simulink model "msl_model"  (R2015a)
settings: configuration reference "config_cosim" (kept outside this file)
model workspace (MATLAB code in the model file):
  | init_msl;
undefined symbols (not defined in the file): Cx, g, Init_beta, Init_epsi, Init_m, Init_psi, Init_R, Init_theta, Init_Vm, Init_Xm, Init_Ym, Init_Zm, Is, N, rou, S
settings Model: Creator=zhang  LastModifiedBy=ericli
settings ConfigSetRef: SourceLocation=Base Workspace

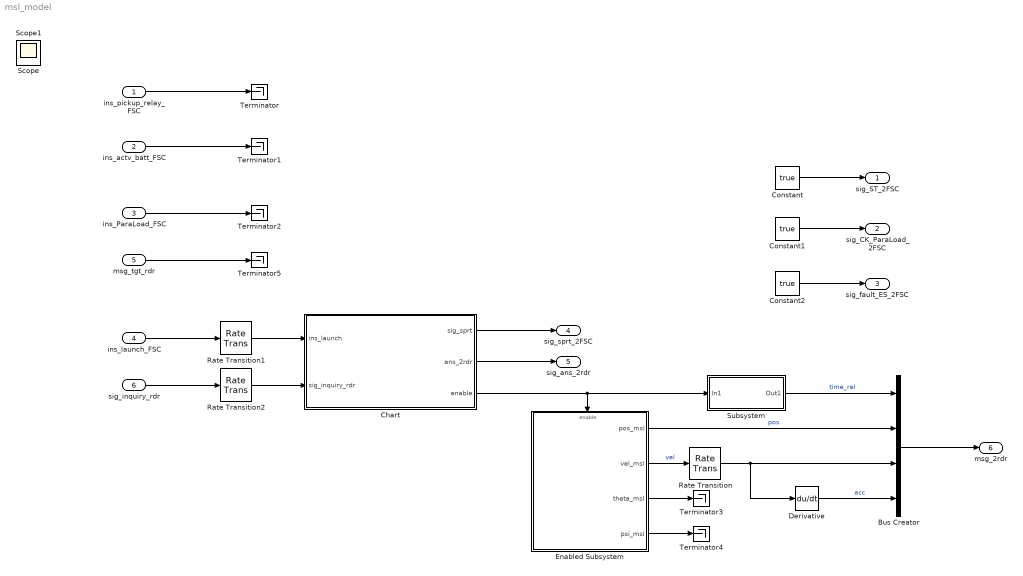
== system msl_model ==
  ins_pickup_relay_FSC : Inport  OutDataTypeStr=boolean
  ins_actv_batt_FSC : Inport  Port=2  OutDataTypeStr=boolean
  ins_ParaLoad_FSC : Inport  Port=3  OutDataTypeStr=boolean
  ins_launch_FSC : Inport  Port=4  OutDataTypeStr=boolean
  msg_tgt_rdr : Inport  Port=5  OutDataTypeStr=Bus: BusObject_msg_rdr2msl  BusOutputAsStruct=on
  sig_inquiry_rdr : Inport  Port=6  OutDataTypeStr=boolean
  Bus Creator : BusCreator  OutDataTypeStr=Bus: BusObject_msg_msl2rdr
      settings: InheritFromInputs=off
  Chart : Stateflow chart  TreatAsAtomicUnit=on
  Constant : Constant  Value=true
  Constant1 : Constant  Value=true
  Constant2 : Constant  Value=true
  Derivative : Derivative
  Enabled Subsystem : Subsystem  TreatAsAtomicUnit=on
  Rate Transition : RateTransition
  Rate Transition1 : RateTransition
  Rate Transition2 : RateTransition
  Subsystem : Subsystem
  Terminator{,1..5} (6 alike) : Terminator
  sig_ST_2FSC : Outport
  sig_CK_ParaLoad_2FSC : Outport  Port=2
  sig_fault_ES_2FSC : Outport  Port=3
  sig_sprt_2FSC : Outport  Port=4
  sig_ans_2rdr : Outport  Port=5
  msg_2rdr : Outport  Port=6  OutDataTypeStr=Bus: BusObject_msg_msl2rdr  BusOutputAsStruct=on
  Scope : Scope  NumInputPorts=3
      settings: YMin=-5~-5~-5  YMax=5~5~5
  Scope1 : Scope  NumInputPorts=3
      settings: YMin=-5~-5~-5  YMax=5~5~5
  wires:
  ins_pickup_relay_FSC/1 -> Terminator/1
  ins_actv_batt_FSC/1 -> Terminator1/1
  ins_ParaLoad_FSC/1 -> Terminator2/1
  ins_launch_FSC/1 -> Rate Transition1/1
  Chart/1(sig_sprt) -> sig_sprt_2FSC/1
  Chart/3(enable) -> Subsystem/1(In1), Enabled Subsystem/Enable
  Enabled Subsystem/4(psi_msl) -> Terminator4/1
  Enabled Subsystem/3(theta_msl) -> Terminator3/1
  Enabled Subsystem/2(vel_msl) -> Rate Transition/1  "vel"
  Constant/1 -> sig_ST_2FSC/1
  Constant1/1 -> sig_CK_ParaLoad_2FSC/1
  Constant2/1 -> sig_fault_ES_2FSC/1
  Chart/2(ans_2rdr) -> sig_ans_2rdr/1
  Enabled Subsystem/1(pos_msl) -> Bus Creator/2  "pos"
  Derivative/1 -> Bus Creator/4  "acc"
  Subsystem/1(Out1) -> Bus Creator/1  "time_rel"
  Bus Creator/1 -> msg_2rdr/1
  msg_tgt_rdr/1 -> Terminator5/1
  sig_inquiry_rdr/1 -> Rate Transition2/1
  Rate Transition/1 -> Derivative/1, Bus Creator/3
  Rate Transition1/1 -> Chart/1(ins_launch)
  Rate Transition2/1 -> Chart/2(sig_inquiry_rdr)

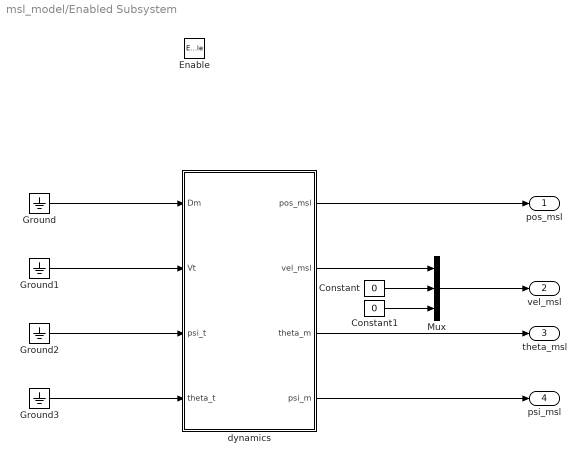
== system msl_model/Enabled Subsystem ==
  Enable : EnablePort
  Constant : Constant  Value=0
  Constant1 : Constant  Value=0
  Ground{,1..3} (4 alike) : Ground
  Mux : Mux  Inputs=3
  dynamics : Subsystem
  pos_msl : Outport
  vel_msl : Outport  Port=2
  theta_msl : Outport  Port=3
  psi_msl : Outport  Port=4
  wires:
  Ground/1 -> dynamics/1(Dm)
  Ground1/1 -> dynamics/2(Vt)
  Ground2/1 -> dynamics/3(psi_t)
  Ground3/1 -> dynamics/4(theta_t)
  dynamics/1(pos_msl) -> pos_msl/1
  dynamics/3(theta_m) -> theta_msl/1
  dynamics/4(psi_m) -> psi_msl/1
  dynamics/2(vel_msl) -> Mux/1
  Mux/1 -> vel_msl/1
  Constant/1 -> Mux/2
  Constant1/1 -> Mux/3

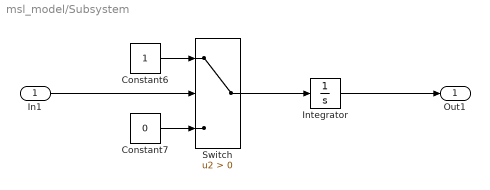
== system msl_model/Subsystem ==
  In1 : Inport
  Constant6 : Constant
  Constant7 : Constant  Value=0
  Integrator : Integrator
  Switch : Switch  Criteria=u2 > Threshold
  Out1 : Outport
  wires:
  Constant7/1 -> Switch/3
  Constant6/1 -> Switch/1
  Switch/1 -> Integrator/1
  Integrator/1 -> Out1/1
  In1/1 -> Switch/2

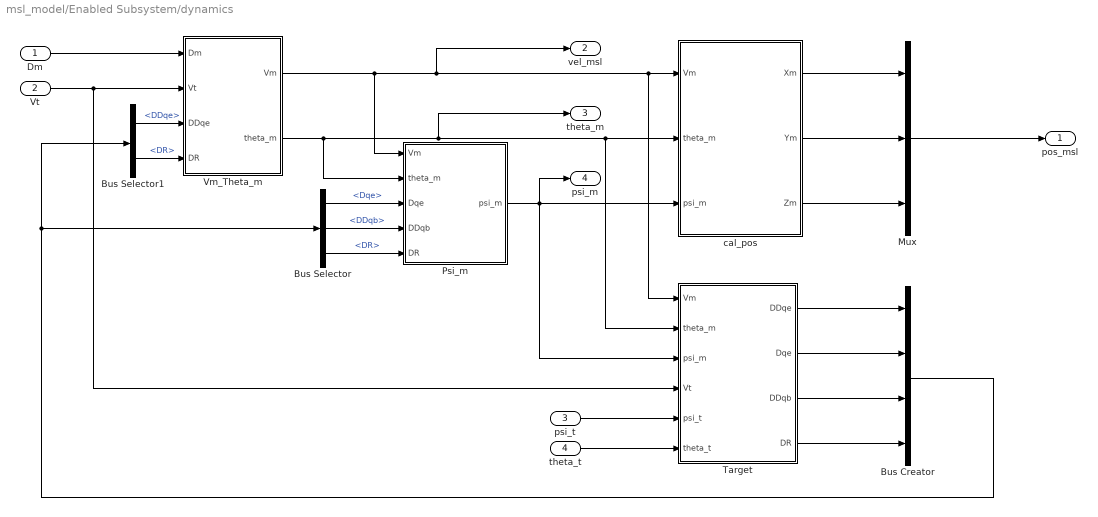
== system msl_model/Enabled Subsystem/dynamics ==
  Dm : Inport
  Vt : Inport  Port=2
  psi_t : Inport  Port=3
  theta_t : Inport  Port=4
  Bus Creator : BusCreator
  Bus Selector : BusSelector  OutputSignals=Dqe,DDqb,DR
  Bus Selector1 : BusSelector  OutputSignals=DDqe,DR
  Mux : Mux  Inputs=3
  Psi_m : Subsystem
  Target : Subsystem
  Vm_Theta_m : Subsystem
  cal_pos : Subsystem
  pos_msl : Outport
  vel_msl : Outport  Port=2
  theta_m : Outport  Port=3
  psi_m : Outport  Port=4
  wires:
  Psi_m/1(psi_m) -> psi_m/1, cal_pos/3(psi_m), Target/3(psi_m)
  Bus Selector/3 -> Psi_m/5(DR)  "<DR>"
  theta_t/1 -> Target/6(theta_t)
  Vt/1 -> Target/4(Vt), Vm_Theta_m/2(Vt)
  Target/2(Dqe) -> Bus Creator/2
  Bus Selector/1 -> Psi_m/3(Dqe)  "<Dqe>"
  Target/4(DR) -> Bus Creator/4
  cal_pos/3(Zm) -> Mux/3
  Mux/1 -> pos_msl/1
  Vm_Theta_m/1(Vm) -> Psi_m/1(Vm), vel_msl/1, cal_pos/1(Vm), Target/1(Vm)
  Bus Selector1/1 -> Vm_Theta_m/3(DDqe)  "<DDqe>"
  Bus Selector1/2 -> Vm_Theta_m/4(DR)  "<DR>"
  cal_pos/2(Ym) -> Mux/2
  Vm_Theta_m/2(theta_m) -> Psi_m/2(theta_m), theta_m/1, cal_pos/2(theta_m), Target/2(theta_m)
  Dm/1 -> Vm_Theta_m/1(Dm)
  Target/1(DDqe) -> Bus Creator/1
  psi_t/1 -> Target/5(psi_t)
  cal_pos/1(Xm) -> Mux/1
  Target/3(DDqb) -> Bus Creator/3
  Bus Selector/2 -> Psi_m/4(DDqb)  "<DDqb>"
  Bus Creator/1 -> Bus Selector/1, Bus Selector1/1

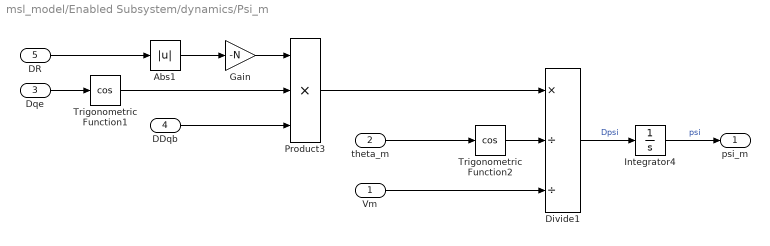
== system msl_model/Enabled Subsystem/dynamics/Psi_m ==
  Vm : Inport
  theta_m : Inport  Port=2
  Dqe : Inport  Port=3
  DDqb : Inport  Port=4
  DR : Inport  Port=5
  Abs1 : Abs
  Divide1 : Product  Inputs=*//
  Gain : Gain  Gain=-N
  Integrator4 : Integrator  InitialCondition=Init_psi
  Product3 : Product  Inputs=3
  Trigonometric Function1 : Trigonometry  Operator=cos
  Trigonometric Function2 : Trigonometry  Operator=cos
  psi_m : Outport
  wires:
  theta_m/1 -> Trigonometric Function2/1
  DR/1 -> Abs1/1
  Vm/1 -> Divide1/3
  Divide1/1 -> Integrator4/1  "Dpsi"
  Integrator4/1 -> psi_m/1  "psi"
  Trigonometric Function2/1 -> Divide1/2
  Dqe/1 -> Trigonometric Function1/1
  Product3/1 -> Divide1/1
  Abs1/1 -> Gain/1
  Gain/1 -> Product3/1
  Trigonometric Function1/1 -> Product3/2
  DDqb/1 -> Product3/3

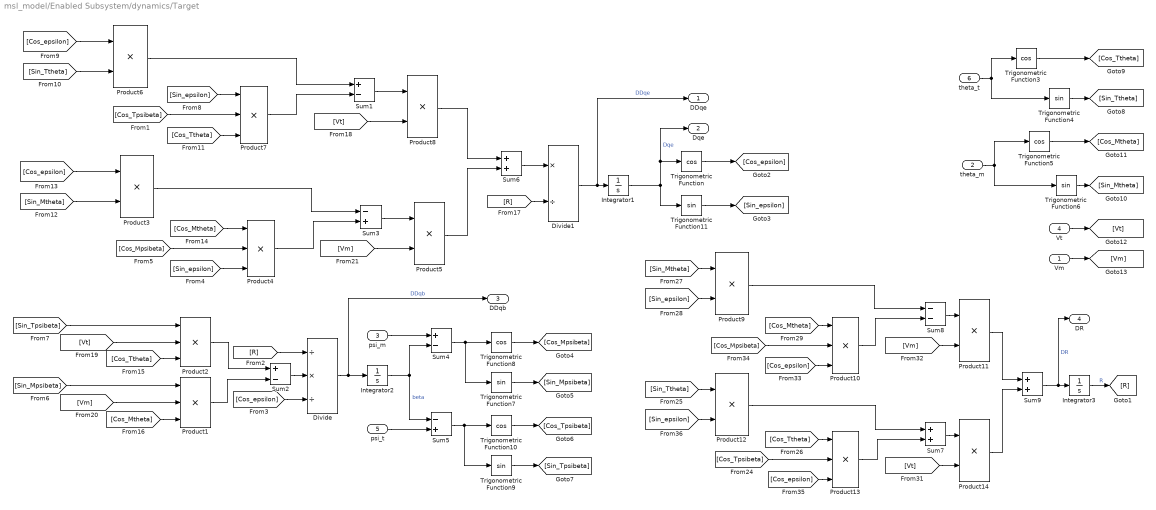
== system msl_model/Enabled Subsystem/dynamics/Target ==
  Vm : Inport
  theta_m : Inport  Port=2
  psi_m : Inport  Port=3
  Vt : Inport  Port=4
  psi_t : Inport  Port=5
  theta_t : Inport  Port=6
  Divide : Product  Inputs=/*/
  Divide1 : Product  Inputs=*/
  Integrator1 : Integrator  InitialCondition=Init_epsi
  Integrator2 : Integrator  InitialCondition=Init_beta
  Integrator3 : Integrator  InitialCondition=Init_R
  Product{1..2,4,7,10,13} (6 alike) : Product  Inputs=3
  Product{3,5..6,8..9,11..12,14} (8 alike) : Product
  Sum1 : Sum  Inputs=+-
  Sum2 : Sum  Inputs=+-
  Sum3 : Sum  Inputs=-+
  Sum4 : Sum  Inputs=+-
  Sum5 : Sum  Inputs=-+
  Sum6 : Sum
  Sum7 : Sum
  Sum8 : Sum  Inputs=--
  Sum9 : Sum
  Trigonometric Function{,3,5,8,10} (5 alike) : Trigonometry  Operator=cos
  Trigonometric Function{4,6..7,9,11} (5 alike) : Trigonometry
  DDqe : Outport
  Dqe : Outport  Port=2
  DDqb : Outport  Port=3
  DR : Outport  Port=4
  wires:
  Integrator1/1 -> Dqe/1, Trigonometric Function/1, Trigonometric Function11/1  "Dqe"
  Divide1/1 -> DDqe/1, Integrator1/1  "DDqe"
  Integrator2/1 -> Sum5/1, Sum4/2  "beta"
  Divide/1 -> DDqb/1, Integrator2/1  "DDqb"
  Integrator3/1 -> [R]  "R"
  Sum9/1 -> DR/1, Integrator3/1  "DR"
  Trigonometric Function/1 -> [Cos_epsilon]
  theta_m/1 -> Trigonometric Function5/1, Trigonometric Function6/1
  Trigonometric Function5/1 -> [Cos_Mtheta]
  Product2/1 -> Sum2/1
  Product1/1 -> Sum2/2
  [Cos_epsilon] -> Divide/3
  Product3/1 -> Sum3/1
  Product4/1 -> Sum3/2
  Sum3/1 -> Product5/1
  Trigonometric Function11/1 -> [Sin_epsilon]
  [Sin_epsilon] -> Product4/3
  psi_m/1 -> Sum4/1
  Sum4/1 -> Trigonometric Function8/1, Trigonometric Function7/1
  Trigonometric Function8/1 -> [Cos_Mpsibeta]
  Trigonometric Function7/1 -> [Sin_Mpsibeta]
  [Cos_Mpsibeta] -> Product4/2
  [Sin_Mpsibeta] -> Product1/1
  Sum5/1 -> Trigonometric Function10/1, Trigonometric Function9/1
  Trigonometric Function10/1 -> [Cos_Tpsibeta]
  Trigonometric Function9/1 -> [Sin_Tpsibeta]
  psi_t/1 -> Sum5/2
  [Sin_Tpsibeta] -> Product2/1
  Trigonometric Function6/1 -> [Sin_Mtheta]
  [Cos_Tpsibeta] -> Product7/2
  [Sin_epsilon] -> Product7/1
  [Cos_epsilon] -> Product6/1
  Product7/1 -> Sum1/2
  Product6/1 -> Sum1/1
  Sum1/1 -> Product8/1
  [Sin_Ttheta] -> Product6/2
  [Cos_Ttheta] -> Product7/3
  [Sin_Mtheta] -> Product3/2
  [Cos_Mtheta] -> Product4/1
  [Cos_Ttheta] -> Product2/3
  [Cos_Mtheta] -> Product1/3
  theta_t/1 -> Trigonometric Function4/1, Trigonometric Function3/1
  Trigonometric Function3/1 -> [Cos_Ttheta]
  Trigonometric Function4/1 -> [Sin_Ttheta]
  [Cos_epsilon] -> Product3/1
  Product5/1 -> Sum6/2
  Product8/1 -> Sum6/1
  Sum6/1 -> Divide1/1
  [R] -> Divide1/2
  Sum2/1 -> Divide/2
  [R] -> Divide/1
  [Vt] -> Product8/2
  [Vt] -> Product2/2
  [Vm] -> Product1/2
  [Vm] -> Product5/2
  Vt/1 -> [Vt]
  Vm/1 -> [Vm]
  Product9/1 -> Sum8/1
  Product10/1 -> Sum8/2
  Sum8/1 -> Product11/1
  [Cos_epsilon] -> Product10/3
  [Cos_Mpsibeta] -> Product10/2
  Product13/1 -> Sum7/2
  Product12/1 -> Sum7/1
  Sum7/1 -> Product14/1
  [Cos_Mtheta] -> Product10/1
  [Vt] -> Product14/2
  [Vm] -> Product11/2
  [Sin_epsilon] -> Product9/2
  [Sin_Mtheta] -> Product9/1
  Product11/1 -> Sum9/1
  Product14/1 -> Sum9/2
  [Sin_Ttheta] -> Product12/1
  [Sin_epsilon] -> Product12/2
  [Cos_Ttheta] -> Product13/1
  [Cos_Tpsibeta] -> Product13/2
  [Cos_epsilon] -> Product13/3

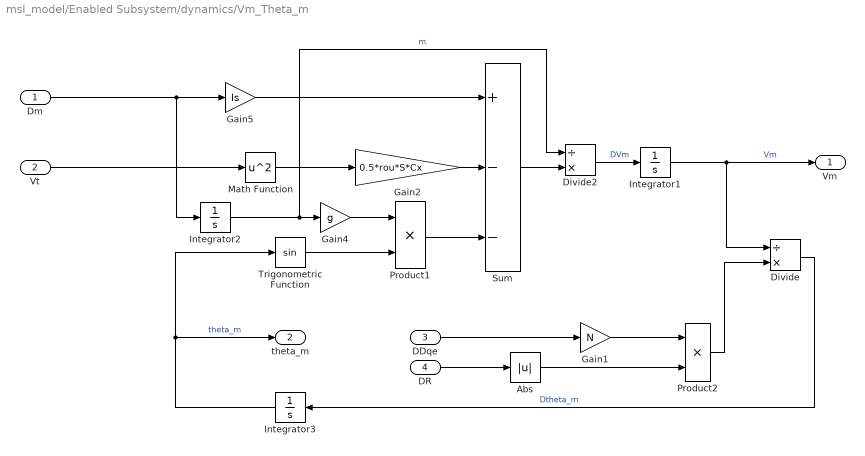
== system msl_model/Enabled Subsystem/dynamics/Vm_Theta_m ==
  Dm : Inport
  Vt : Inport  Port=2
  DDqe : Inport  Port=3
  DR : Inport  Port=4
  Abs : Abs
  Divide : Product  Inputs=/*
  Divide2 : Product  Inputs=/*
  Gain1 : Gain  Gain=N
  Gain2 : Gain  Gain=0.5*rou*S*Cx
  Gain4 : Gain  Gain=g
  Gain5 : Gain  Gain=Is
  Integrator1 : Integrator  InitialCondition=Init_Vm
  Integrator2 : Integrator  InitialCondition=Init_m
  Integrator3 : Integrator  InitialCondition=Init_theta
  Math Function : Math  Operator=square  SaturateOnIntegerOverflow=on
  Product1 : Product
  Product2 : Product
  Sum : Sum  Inputs=+--
  Trigonometric Function : Trigonometry
  Vm : Outport
  theta_m : Outport  Port=2
  wires:
  DDqe/1 -> Gain1/1
  Gain1/1 -> Product2/1
  Integrator1/1 -> Vm/1, Divide/1  "Vm"
  Vt/1 -> Math Function/1
  Gain2/1 -> Sum/2
  Math Function/1 -> Gain2/1
  Gain4/1 -> Product1/1
  Trigonometric Function/1 -> Product1/2
  Dm/1 -> Gain5/1, Integrator2/1
  Gain5/1 -> Sum/1
  Integrator2/1 -> Divide2/1, Gain4/1  "m"
  Product1/1 -> Sum/3
  Sum/1 -> Divide2/2
  Divide2/1 -> Integrator1/1  "DVm"
  Integrator3/1 -> Trigonometric Function/1, theta_m/1  "theta_m"
  Divide/1 -> Integrator3/1  "Dtheta_m"
  DR/1 -> Abs/1
  Abs/1 -> Product2/2
  Product2/1 -> Divide/2

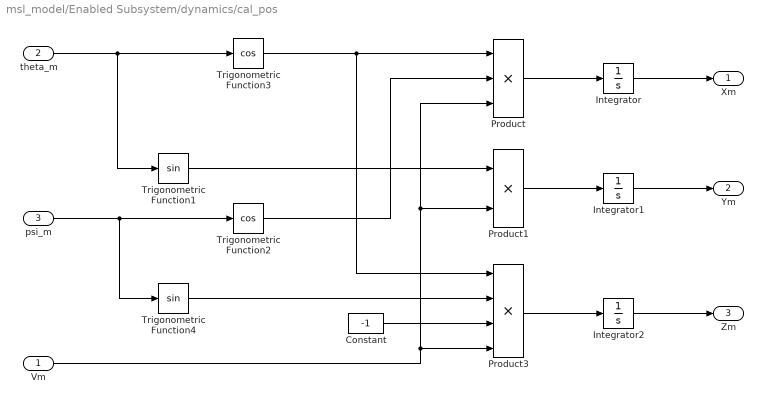
== system msl_model/Enabled Subsystem/dynamics/cal_pos ==
  Vm : Inport
  theta_m : Inport  Port=2
  psi_m : Inport  Port=3
  Constant : Constant  Value=-1
  Integrator : Integrator  InitialCondition=Init_Xm
  Integrator1 : Integrator  InitialCondition=Init_Ym
  Integrator2 : Integrator  InitialCondition=Init_Zm
  Product : Product  Inputs=3
  Product1 : Product
  Product3 : Product  Inputs=4
  Trigonometric Function1 : Trigonometry
  Trigonometric Function2 : Trigonometry  Operator=cos
  Trigonometric Function3 : Trigonometry  Operator=cos
  Trigonometric Function4 : Trigonometry
  Xm : Outport
  Ym : Outport  Port=2
  Zm : Outport  Port=3
  wires:
  Product3/1 -> Integrator2/1
  Trigonometric Function4/1 -> Product3/2
  Trigonometric Function1/1 -> Product1/1
  Product/1 -> Integrator/1
  Trigonometric Function2/1 -> Product/2
  Trigonometric Function3/1 -> Product3/1, Product/1
  Constant/1 -> Product3/3
  Product1/1 -> Integrator1/1
  Vm/1 -> Product1/2, Product/3, Product3/4
  psi_m/1 -> Trigonometric Function2/1, Trigonometric Function4/1
  theta_m/1 -> Trigonometric Function1/1, Trigonometric Function3/1
  Integrator2/1 -> Zm/1
  Integrator1/1 -> Ym/1
  Integrator/1 -> Xm/1

== stateflow chart msl_model/Chart ==
  state prepare
  state launch
    en: enable = true;
  state flight
    en:
    enable = true;
    sig_sprt = true;
    (default) -> (junction 10)
    (junction 10) -> (junction 12) [order 1] : [sig_inquiry_rdr]
    (junction 10) -> (junction 16) [order 2]
    (junction 12) -> (junction 14) : {
        | ans_2rdr = true;
        | }
    (junction 14) -> (junction 16)
  (default) -> prepare : {
      | enable = false;
      | }
  prepare -> launch : [ins_launch]
  launch -> flight : after(0.2,sec)
  data: ins_launch input boolean; sig_sprt output boolean; ans_2rdr output boolean; enable output boolean; sig_inquiry_rdr input boolean
